simulink model "AHRS_voter_Harness_SLDV"  (R2019a)
settings: Solver=FixedStepDiscrete  StartTime=0  StopTime=0.01  FixedStep=0.01  RelTol=1e-3  EnableMultiTasking=on
Description:
  | Test harness for SLDV generated test cases.
settings Model: DataDictionary=HeliSystemDD.sldd  Creator=bpotter  LastModifiedBy=bpotter
settings DataIOCC: LimitDataPoints=on  ReturnWorkspaceOutputs=off
settings OptimizationCC: BlockReduction=off  ConditionallyExecuteInputs=off  DefaultParameterBehavior=Inlined  UseDivisionForNetSlopeComputation=on  ExpressionFolding=off  InitFltsAndDblsToZero=on  EfficientFloat2IntCast=on  EfficientMapNaN2IntZero=off  LifeSpan=inf  MaxStackSize=inf
settings DebuggingCC: SignalInfNanChecking=error  SignalRangeChecking=error  ReadBeforeWriteMsg=EnableAllAsError  WriteAfterWriteMsg=EnableAllAsError  WriteAfterReadMsg=EnableAllAsError  AlgebraicLoopMsg=error  ArtificialAlgebraicLoopMsg=error  SaveWithDisabledLinksMsg=error  SaveWithParameterizedLinksMsg=error  BlockPriorityViolationMsg=error  SolverPrmCheckMsg=error  InheritedTsInSrcMsg=none  SingleTaskRateTransMsg=error  TasksWithSamePriorityMsg=error  SigSpecEnsureSampleTimeMsg=error  CheckMatrixSingularityMsg=error  IntegerOverflowMsg=error  ParameterUnderflowMsg=error  ParameterPrecisionLossMsg=error  ParameterTunabilityLossMsg=error  UnderSpecifiedDataTypeMsg=error  UnnecessaryDatatypeConvMsg=warning  VectorMatrixConversionMsg=error  SignalLabelMismatchMsg=error  UnconnectedInputMsg=error  UnconnectedOutputMsg=error  UnconnectedLineMsg=error  SFcnCompatibilityMsg=error  UniqueDataStoreMsg=error  BusObjectLabelMismatch=error  RootOutportRequireBusObject=error  AssertControl=DisableAll  AllowSymbolicDim=off  ModelReferenceIOMsg=error  ModelReferenceIOMismatchMessage=error  UnknownTsInhSupMsg=error  ModelReferenceDataLoggingMessage=error  StateNameClashWarn=warning  PregeneratedLibrarySubsystemCodeDiagnostic=none  StrictBusMsg=ErrorOnBusTreatedAsVector  NonBusSignalsTreatedAsBus=error  SFInvalidInputDataAccessInChartInitDiag=error  SFTransitionOutsideNaturalParentDiag=error  SFUnreachableExecutionPathDiag=error  SFUndirectedBroadcastEventsDiag=error  SFTransitionActionBeforeConditionDiag=error  SFExecutionAtInitializationDiag=none  IntegerSaturationMsg=error  ArithmeticOperatorsInVariantConditions=warning
settings HardwareCC: ProdBitPerPointer=32  ProdBitPerSizeT=32  ProdBitPerPtrDiffT=32  ProdWordSize=32  ProdHWDeviceType=Intel->x86-32 (Windows32)  TargetIntDivRoundTo=Zero
settings ModelReferenceCC: ModelReferenceNumInstancesAllowed=Single  PropagateSignalLabelsOutOfModel=off
settings SFSimCC: SimUseLocalCustomCode=off  CompileTimeRecursionLimit=0  EnableRuntimeRecursion=off  MATLABDynamicMemAlloc=off
settings RTWCC: SystemTargetFile=ert.tlc  TemplateMakefile=ert_default_tmf  GenerateReport=on  RTWUseLocalCustomCode=off  IncludeHyperlinkInReport=on  LaunchReport=on  PortableWordSizes=on  GenerateTraceInfo=on  GenerateTraceReport=on  GenerateTraceReportSl=on  GenerateTraceReportSf=on  GenerateTraceReportEml=on
settings CodeAppCC: ForceParamTrailComments=on  IgnoreCustomStorageClasses=off  MATLABFcnDesc=on  MangleLength=4  StateflowObjectComments=on  ReqsInCode=on
settings ERTTargetCC: TargetLangStandard=C99 (ISO)  UtilityFuncGeneration=Shared location  MultiwordLength=2048  GenerateSampleERTMain=on  IncludeMdlTerminateFcn=off  SuppressErrorStatus=on  SupportAbsoluteTime=off  SupportNonFinite=off  ParenthesesLevel=Maximum  CastingMode=Standards  GenerateSharedConstants=off  ERTCustomFileTemplate=example_file_process.tlc  ERTFilePackagingFormat=Compact  PreserveExpressionOrder=on  PreserveIfCondition=on  ConvertIfToSwitch=off  SuppressUnreachableDefaultCases=off  EnableSignedLeftShifts=off  EnableSignedRightShifts=off
settings ConfigComp: CovEnable=on  CovScope=ReferencedModels  CovIncludeTopModel=off  CovMetricSettings=dcmobe  CovHTMLOptions=-aTS=1 -bRG=1 -bTC=0 -hTR=0 -nFC=0 -scm=1 -bcm=1  CovHtmlReporting=on  CovSaveCumulativeToWorkspaceVar=on  CovCumulativeVarName=AHRScovCumData  CovCumulativeReport=on  CovModelRefEnable=on  PSVerificationMode=BugFinder  PSResultDir=\BugFinder_results  PSModelRefVerifDepth=All  PSAutoStubLUT=off  DVMakeOutputFilesUnique=off  DVModelCoverageObjectives=MCDC  DVTestSuiteOptimization=IndividualObjectives  DVIgnoreCovSatisfied=on  DVCoverageDataFile=simulation_results\AHRS_voter_cov.cvt  DVIncludeRelationalBoundary=on  DVSaveDataFile=off  DVSaveReport=on  DVReportPDFFormat=on  DVRebuildModelRepresentation=Always

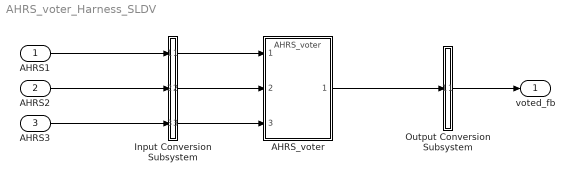
== system AHRS_voter_Harness_SLDV ==
  AHRS1 : Inport  OutDataTypeStr=Bus: AHRS_Bus  PortDimensions=[1]  SampleTime=0.01  Interpolate=off  BusOutputAsStruct=on
  AHRS2 : Inport  Port=2  OutDataTypeStr=Bus: AHRS_Bus  PortDimensions=[1]  SampleTime=0.01  Interpolate=off  BusOutputAsStruct=on
  AHRS3 : Inport  Port=3  OutDataTypeStr=Bus: AHRS_Bus  PortDimensions=[1]  SampleTime=0.01  Interpolate=off  BusOutputAsStruct=on
  AHRS_voter : ModelReference  ModelNameDialog=AHRS_voter  SimulationMode=Normal  ModelReferenceVersion=1.64
  Input Conversion Subsystem : Subsystem  Tag=__SLT_ICS__  Description=|
      | Signal spec.
      | and routing
      settings: AttributesFormatString=%<Description>
  Output Conversion Subsystem : Subsystem  Tag=__SLT_OCS__  Description=|
      | Signal spec.
      | and routing
      settings: AttributesFormatString=%<Description>
  voted_fb : Outport  OutDataTypeStr=double  PortDimensions=[5]
  wires:
  AHRS1/1 -> Input Conversion Subsystem/1(Inport_1)
  AHRS2/1 -> Input Conversion Subsystem/2(Inport_2)
  AHRS3/1 -> Input Conversion Subsystem/3(Inport_3)
  Output Conversion Subsystem/1(Outport_1) -> voted_fb/1
  Input Conversion Subsystem/1(Outport_1) -> AHRS_voter/1
  Input Conversion Subsystem/2(Outport_2) -> AHRS_voter/2
  Input Conversion Subsystem/3(Outport_3) -> AHRS_voter/3
  AHRS_voter/1 -> Output Conversion Subsystem/1(Inport_1)

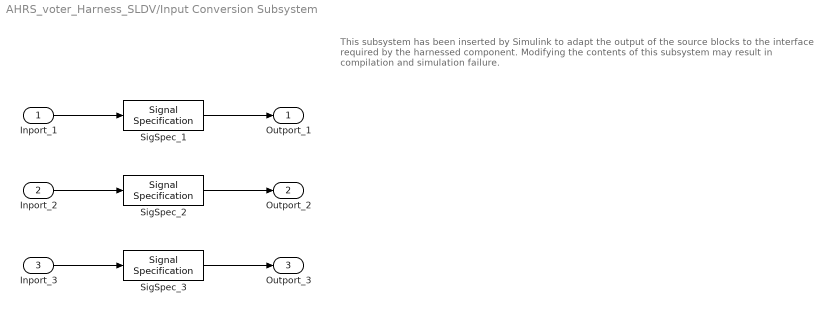
== system AHRS_voter_Harness_SLDV/Input Conversion Subsystem ==
  note: This subsystem has been inserted by Simulink to adapt the output of the source blocks to the interface required by the harnessed component.
      |  Modifying the contents of this subsystem may result in compilation and simulation failure.
  Inport_1 : Inport
  Inport_2 : Inport  Port=2
  Inport_3 : Inport  Port=3
  SigSpec_1 : SignalSpecification  OutDataTypeStr=Bus: AHRS_Bus  Dimensions=[1]  SampleTime=0.01  BusOutputAsStruct=on
  SigSpec_2 : SignalSpecification  OutDataTypeStr=Bus: AHRS_Bus  Dimensions=[1]  SampleTime=0.01  BusOutputAsStruct=on
  SigSpec_3 : SignalSpecification  OutDataTypeStr=Bus: AHRS_Bus  Dimensions=[1]  SampleTime=0.01  BusOutputAsStruct=on
  Outport_1 : Outport
  Outport_2 : Outport  Port=2
  Outport_3 : Outport  Port=3
  wires:
  SigSpec_1/1 -> Outport_1/1
  Inport_1/1 -> SigSpec_1/1
  SigSpec_2/1 -> Outport_2/1
  Inport_2/1 -> SigSpec_2/1
  SigSpec_3/1 -> Outport_3/1
  Inport_3/1 -> SigSpec_3/1

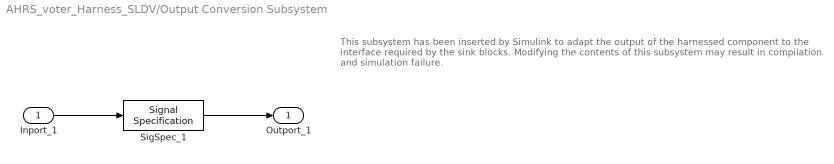
== system AHRS_voter_Harness_SLDV/Output Conversion Subsystem ==
  note: This subsystem has been inserted by Simulink to adapt the output of the harnessed component to the interface required by the sink blocks.
      |  Modifying the contents of this subsystem may result in compilation and simulation failure.
  Inport_1 : Inport
  SigSpec_1 : SignalSpecification  OutDataTypeStr=double  Dimensions=[5]  SampleTime=0.01
  Outport_1 : Outport
  wires:
  Inport_1/1 -> SigSpec_1/1
  SigSpec_1/1 -> Outport_1/1
